simulink model "Mech_473_Projectreport"  (R2017a)
settings: Solver=VariableStepAuto  StartTime=0.0  StopTime=1  RelTol=1e-3
settings Model: Creator=ni_daly  LastModifiedBy=ni_daly

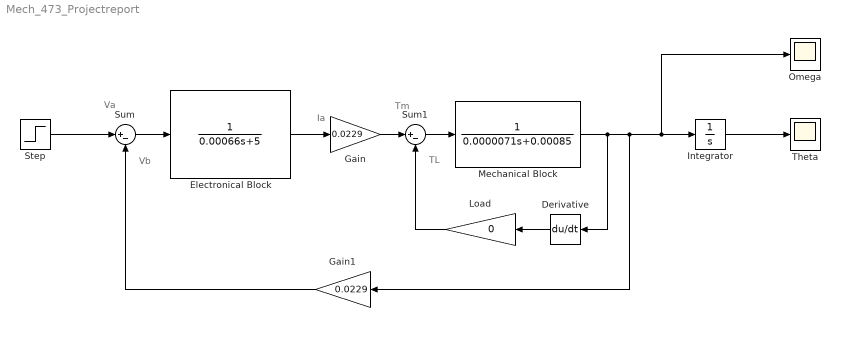
== system Mech_473_Projectreport ==
  note: TL
  note: Tm
  note: Ia
  note: Vb
  note: Va
  Derivative : Derivative
  Electronical Block : TransferFcn  Denominator=[0.00066 5]
  Gain : Gain  Gain=0.0229
  Gain1 : Gain  Gain=0.0229
  Integrator : Integrator
  Load : Gain  Gain=0
  Mechanical Block : TransferFcn  Denominator=[0.0000071 0.00085]
  Omega : Scope
  Step : Step  Time=0.1  SampleTime=0
  Sum : Sum  Inputs=|+-
  Sum1 : Sum  Inputs=|+-
  Theta : Scope
  wires:
  Sum/1 -> Electronical Block/1
  Electronical Block/1 -> Gain/1
  Gain/1 -> Sum1/1
  Sum1/1 -> Mechanical Block/1
  Mechanical Block/1 -> Derivative/1, Gain1/1, Omega/1, Integrator/1
  Integrator/1 -> Theta/1
  Gain1/1 -> Sum/2
  Step/1 -> Sum/1
  Derivative/1 -> Load/1
  Load/1 -> Sum1/2
